simulink model "fft32kpt_ssr16_fixed"  (R2024b)
settings: Solver=VariableStepAuto  StartTime=0.0  StopTime=sample_period*N*5  RelTol=1e-3
PreLoadFcn:
  | clk_freq = 570e6; % PL clock frequency
  | sample_period = 1/(570e6*16); % 570Msps*16parallel paths
  | N=32768; % fft point size
  | binw=(1/sample_period) / 2*N; % bin width
  | 
  | bin_freq = 2*pi*11*binw+pi*binw; % sin, cos freq centering per channel
  | 
  | % for transpose block
  | DATA_WIDTH=16;
  | SSR=16;
  | M=16;
  | N1=N/M;
  | MEM_STYLE=4; % MEM OPTIONS: 4 - ULTRA, 0 - AUTO, 1 - BRAM, 5 - MIXED
InitFcn:
  | clk_freq = 570e6; % PL clock frequency
  | sample_period = 1/(570e6*16); % 570Msps*16parallel paths
  | N=32768; % fft point size
  | binw=(1/sample_period) / 2*N; % bin width
  | 
  | bin_freq = 2*pi*11*binw+pi*binw; % sin, cos freq centering per channel
  | 
  | % for transpose block
  | DATA_WIDTH=16;
  | SSR=16;
  | M=16;
  | N1=N/M;
  | MEM_STYLE=4; % MEM OPTIONS: 4 - ULTRA, 0 - AUTO, 1 - BRAM, 5 - MIXED
undefined symbols (not defined in the file or in its folder): None, S, vsva2197, xcvc1902
libraries: aieBasic x47, hdlBasic x39, aieUtilities x16, aieDSP x16, hdlUtilities x16, matrix_library x16, hdlSSR x13, simulink x1, dspxfrm3 x1, vmcUtilities x1
(part 3 of 3)

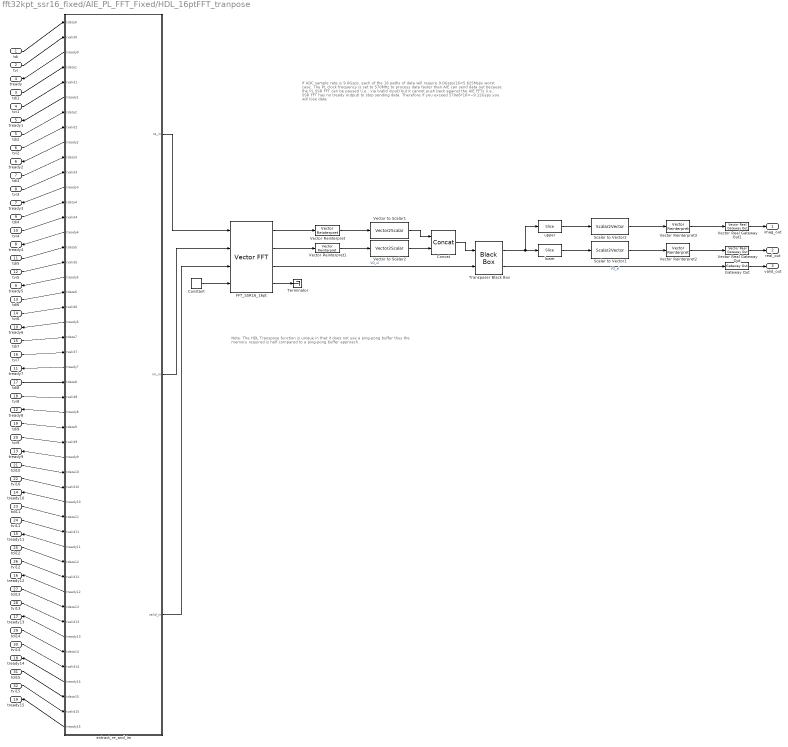
== system fft32kpt_ssr16_fixed/AIE_PL_FFT_Fixed/HDL_16ptFFT_tranpose ==
  note: If ADC sample rate is 9.0Gsps, each of the 16 paths of data will require 9.0Gsps/16=5.625Msps worst case. The PL clock frequency is set to 570MHz to process data faster than AIE can send data out because the PL SSR FFT can be paused (i.e.: via tvalid input) but it cannot push back against the AIE FFTs (i.e.: SSR FFT has no tready output) to stop sending data. Therefore if you exceed 570e6*16=~9.12Gsps you will lose data
  note: Note: The HDL Transpose function is unique in that it does not use a ping-pong buffer thus the memory required is half compared to a ping-pong buffer approach.
  tdi : Inport
  tvi : Inport  Port=2
  tdi1 : Inport  Port=3
  tvi1 : Inport  Port=4
  tdi2 : Inport  Port=5
  tvi2 : Inport  Port=6
  tdi3 : Inport  Port=7
  tvi3 : Inport  Port=8
  tdi4 : Inport  Port=9
  tvi4 : Inport  Port=10
  tdi5 : Inport  Port=11
  tvi5 : Inport  Port=12
  tdi6 : Inport  Port=13
  tvi6 : Inport  Port=14
  tdi7 : Inport  Port=15
  tvi7 : Inport  Port=16
  tdi8 : Inport  Port=17
  tvi8 : Inport  Port=18
  tdi9 : Inport  Port=19
  tvi9 : Inport  Port=20
  tdi10 : Inport  Port=21
  tvi10 : Inport  Port=22
  tdi11 : Inport  Port=23
  tvi11 : Inport  Port=24
  tdi12 : Inport  Port=25
  tvi12 : Inport  Port=26
  tdi13 : Inport  Port=27
  tvi13 : Inport  Port=28
  tdi14 : Inport  Port=29
  tvi14 : Inport  Port=30
  tdi15 : Inport  Port=31
  tvi15 : Inport  Port=32
  Concat : hdlBasic/Concat  num_inputs=2  XmcBlockStatus=1  maskContainerNames=group1  block_type=concat  block_config=sysgen:Concat_config
  Constant : hdlBasic/Constant  const=15  gui_display_data_type=Fixed-point  arith_type=Unsigned  n_bits=log2(16)  bin_pt=0  preci_type=Single  exp_width=8  frac_width=24  explicit_period=on  period=1/clk_freq  XmcBlockStatus=1  maskContainerNames=tabcontainer1  block_type=constant  block_config=sysgen:Constant_config
  FFT_SSR16_16pt : hdlSSR/Vector FFT  N=16  n_bits=16  bin_pt=0  rounding=on  bypass_input_swap=off  bypass_ouput_dsn=off  bram_threshold=258  use_cm4=3  use_cb=on  sg_ssr=16  block_type=fft_ssr  W_high=1  W_low=-17  XmcBlockStatus=1  sg_ssr_prev=16  maskContainerNames=group3
  Gateway Out : hdlBasic/Gateway Out  inherit_from_input=off  bool_to_boolean=off  hdl_port=on  rows=1  columns=1  UseAsDAC=off  DACChannel='1'  interface=None  automatic_assignment=on  address_offset=hex2dec('00')  intf_name=''  intf_description=''  timing_constraint=None  locs_specified=off  LOCs={}  io_standard={}  XmcBlockStatus=1  maskContainerNames=group4  block_type=gatewayout  block_config=sysgen:gateway_out_config  block_width_w=590  block_height_w=620  block_width=620  block_height=750
  Scalar to Vector1 : hdlSSR/Scalar2Vector  Width=DATA_WIDTH  sg_ssr=SSR  block_type=scalar2vector_ssr  XmcBlockStatus=1  sg_ssr_prev=16  maskContainerNames=group1
  Scalar to Vector2 : hdlSSR/Scalar2Vector  Width=DATA_WIDTH  sg_ssr=SSR  block_type=scalar2vector_ssr  XmcBlockStatus=1  sg_ssr_prev=16  maskContainerNames=group1
  Terminator : Terminator
  Transposer Black Box : hdlBasic/Black Box  init_code=ssr_transpose_top_config  sim_method=Vivado Simulator  engine_block=../../Questa  verbose=on  XmcBlockStatus=1  maskContainerNames=group1  block_type=blackbox2  block_config=sysgen:black_box_config
  Vector Real Gateway Out : hdlSSR/Vector Real Gateway Out  inherit_from_input=off  hdl_port=on  sg_ssr=16  rows=1  columns=1  UseAsDAC=off  DACChannel='1'  interface=None  automatic_assignment=on  address_offset=hex2dec('00')  intf_name=''  intf_description=''  timing_constraint=None  locs_specified=off  LOCs={}  io_standard={}  block_type=realgatewayout_ssr  XmcBlockStatus=1  sg_ssr_prev=16  maskContainerNames=group4  block_width_w=590  block_height_w=620  block_width=620  block_height=750
  Vector Real Gateway Out1 : hdlSSR/Vector Real Gateway Out  inherit_from_input=off  hdl_port=on  sg_ssr=16  rows=1  columns=1  UseAsDAC=off  DACChannel='1'  interface=None  automatic_assignment=on  address_offset=hex2dec('00')  intf_name=''  intf_description=''  timing_constraint=None  locs_specified=off  LOCs={}  io_standard={}  block_type=realgatewayout_ssr  XmcBlockStatus=1  sg_ssr_prev=16  maskContainerNames=group4  block_width_w=590  block_height_w=620  block_width=620  block_height=750
  Vector Reinterpret : hdlSSR/Vector Reinterpret  force_arith_type=on  arith_type=Unsigned  force_bin_pt=on  bin_pt=0  sg_ssr=SSR  block_type=reinterpret_ssr  XmcBlockStatus=1  sg_ssr_prev=16  maskContainerNames=group1
  Vector Reinterpret1 : hdlSSR/Vector Reinterpret  force_arith_type=on  arith_type=Unsigned  force_bin_pt=on  bin_pt=0  sg_ssr=SSR  block_type=reinterpret_ssr  XmcBlockStatus=1  sg_ssr_prev=16  maskContainerNames=group1
  Vector Reinterpret2 : hdlSSR/Vector Reinterpret  force_arith_type=on  arith_type="Signed  (2's comp)"  force_bin_pt=off  bin_pt=0  sg_ssr=SSR  block_type=reinterpret_ssr  XmcBlockStatus=1  sg_ssr_prev=16  maskContainerNames=group1
  Vector Reinterpret3 : hdlSSR/Vector Reinterpret  force_arith_type=on  arith_type="Signed  (2's comp)"  force_bin_pt=off  bin_pt=0  sg_ssr=SSR  block_type=reinterpret_ssr  XmcBlockStatus=1  sg_ssr_prev=16  maskContainerNames=group1
  Vector to Scalar1 : hdlSSR/Vector2Scalar  sg_ssr=SSR  block_type=vector2scalar_ssr  XmcBlockStatus=1  sg_ssr_prev=16  maskContainerNames=group1
  Vector to Scalar2 : hdlSSR/Vector2Scalar  sg_ssr=SSR  block_type=vector2scalar_ssr  XmcBlockStatus=1  sg_ssr_prev=16  maskContainerNames=group1
  extract_re_and_im : Subsystem
      settings: PortSchema="{\"entries\":[{\"content\":{\"sides\":[{\"content\":{\"connectorIds\":[\"In1\",\"In2\",\"Out4\",\"In3\",\"In4\",\"Out5\",\"In5\",\"In6\",\"Out6\",\"In7\",\"In8\",\"Out7\",\"In9\",\"In10\",\"Out8\",\"In11\",\"In12\",\"Out9\",\"In13\",\"In14\",\"Out10\",\"In15\",\"In16\",\"Out11\",\"In17\",\"In18\",\"Out12\",\"In19\",\"In20\",\"Out13\",\"In21\",\"In22\",\"Out14\",\"In23\",\"In24\",\"Out15\",\"In25\",\"In26\",\"Out16\",\"In27\",\"In28\",\"Out17\",\"In29\",\"In30\",\"Out18\",\"In31\",\"In32\",\"Out19\"]},\"type\":\"ConnectorPlacement.EquallySpacedRectSide\",\"uuid\":\"4c9cd091-c59a-490e-903e-02f0ef96851d\"},{\"content\":{\"connectorIds\":[\"Out1\",\"Out2\",\"Out3\"],\"side\":\"RIGHT\"},\"type\":\"ConnectorPlacement.EquallySpacedRectSide\",\"uuid\":\"c05feb9a-4f35-4110-be75-dac51685fe1e\"},{\"content\":{\"side\":\"TOP\"},\"type\":\"ConnectorPlacement.EquallySpacedRectSide\",\"uuid\":\"aa818d08-a3bb-44ec-b82c-f7b75f0c5c84\"}]},\"type\":\"ConnectorPlacement.EquallySpacedConnector\",\"uuid\":\"837a6877-8b4b-4e86-8a21-a8261c1d8bd7\"}],\"packageUris\":[\"http://schema.mathworks.com/mf0/Connector/R2020b\"],\"version\":\"1.0\"}"
  lower : hdlBasic/Slice  nbits=DATA_WIDTH*SSR  boolean_output=off  mode=Lower Bit Location + Width  bit1=0  base1=MSB of Input  bit0=0  base0=LSB of Input  XmcBlockStatus=1  maskContainerNames=group1  block_type=slice  block_config=sysgen:Slice_config
  upper : hdlBasic/Slice  nbits=DATA_WIDTH*SSR  boolean_output=off  mode=Upper Bit Location + Width  bit1=0  base1=MSB of Input  bit0=0  base0=LSB of Input  XmcBlockStatus=1  maskContainerNames=group1  block_type=slice  block_config=sysgen:Slice_config
  imag_out : Outport
  real_out : Outport  Port=2
  valid_out : Outport  Port=3
  tready : Outport  Port=4
  tready1 : Outport  Port=5
  tready2 : Outport  Port=6
  tready3 : Outport  Port=7
  tready4 : Outport  Port=8
  tready5 : Outport  Port=9
  tready6 : Outport  Port=10
  tready7 : Outport  Port=11
  tready8 : Outport  Port=12
  tready9 : Outport  Port=13
  tready10 : Outport  Port=14
  tready11 : Outport  Port=15
  tready12 : Outport  Port=16
  tready13 : Outport  Port=17
  tready14 : Outport  Port=18
  tready15 : Outport  Port=19
  wires:
  FFT_SSR16_16pt/4 -> Terminator/1
  Constant/1 -> FFT_SSR16_16pt/4
  extract_re_and_im/1(re_in) -> FFT_SSR16_16pt/1
  extract_re_and_im/2(im_in) -> FFT_SSR16_16pt/2
  tdi/1 -> extract_re_and_im/1(tdata0)
  tvi/1 -> extract_re_and_im/2(tvalid0)
  tdi1/1 -> extract_re_and_im/3(tdata1)
  tvi1/1 -> extract_re_and_im/4(tvalid1)
  tdi2/1 -> extract_re_and_im/5(tdata2)
  tvi2/1 -> extract_re_and_im/6(tvalid2)
  tdi3/1 -> extract_re_and_im/7(tdata3)
  tvi3/1 -> extract_re_and_im/8(tvalid3)
  tdi4/1 -> extract_re_and_im/9(tdata4)
  tvi4/1 -> extract_re_and_im/10(tvalid4)
  tdi5/1 -> extract_re_and_im/11(tdata5)
  tvi5/1 -> extract_re_and_im/12(tvalid5)
  tdi6/1 -> extract_re_and_im/13(tdata6)
  tvi6/1 -> extract_re_and_im/14(tvalid6)
  tdi7/1 -> extract_re_and_im/15(tdata7)
  tvi7/1 -> extract_re_and_im/16(tvalid7)
  tdi8/1 -> extract_re_and_im/17(tdata8)
  tvi8/1 -> extract_re_and_im/18(tvalid8)
  tdi9/1 -> extract_re_and_im/19(tdata9)
  tvi9/1 -> extract_re_and_im/20(tvalid9)
  tdi10/1 -> extract_re_and_im/21(tdata10)
  tvi10/1 -> extract_re_and_im/22(tvalid10)
  tdi11/1 -> extract_re_and_im/23(tdata11)
  tvi11/1 -> extract_re_and_im/24(tvalid11)
  tdi12/1 -> extract_re_and_im/25(tdata12)
  tvi12/1 -> extract_re_and_im/26(tvalid12)
  tdi13/1 -> extract_re_and_im/27(tdata13)
  tvi13/1 -> extract_re_and_im/28(tvalid13)
  tdi14/1 -> extract_re_and_im/29(tdata14)
  tvi14/1 -> extract_re_and_im/30(tvalid14)
  tdi15/1 -> extract_re_and_im/31(tdata15)
  tvi15/1 -> extract_re_and_im/32(tvalid15)
  extract_re_and_im/4(tready0) -> tready/1
  extract_re_and_im/5(tready1) -> tready1/1
  extract_re_and_im/6(tready2) -> tready2/1
  extract_re_and_im/3(valid_in) -> FFT_SSR16_16pt/3
  extract_re_and_im/7(tready3) -> tready3/1
  extract_re_and_im/8(tready4) -> tready4/1
  extract_re_and_im/9(tready5) -> tready5/1
  extract_re_and_im/10(tready6) -> tready6/1
  extract_re_and_im/11(tready7) -> tready7/1
  extract_re_and_im/12(tready8) -> tready8/1
  extract_re_and_im/13(tready9) -> tready9/1
  extract_re_and_im/14(tready10) -> tready10/1
  extract_re_and_im/15(tready11) -> tready11/1
  extract_re_and_im/16(tready12) -> tready12/1
  extract_re_and_im/17(tready13) -> tready13/1
  extract_re_and_im/18(tready14) -> tready14/1
  extract_re_and_im/19(tready15) -> tready15/1
  FFT_SSR16_16pt/2 -> Vector Reinterpret1/1
  FFT_SSR16_16pt/1 -> Vector Reinterpret/1
  FFT_SSR16_16pt/3 -> Transposer Black Box/2  "VO_sl"
  Vector Reinterpret2/1 -> Vector Real Gateway Out/1
  Vector Reinterpret3/1 -> Vector Real Gateway Out1/1
  Transposer Black Box/2 -> Gateway Out/1  "VO_sl"
  Vector to Scalar1/1 -> Concat/1
  Vector Reinterpret/1 -> Vector to Scalar1/1
  Scalar to Vector1/1 -> Vector Reinterpret2/1
  Transposer Black Box/1 -> upper/1, lower/1
  Vector to Scalar2/1 -> Concat/2
  lower/1 -> Scalar to Vector1/1
  Concat/1 -> Transposer Black Box/1
  upper/1 -> Scalar to Vector2/1
  Vector Reinterpret1/1 -> Vector to Scalar2/1
  Scalar to Vector2/1 -> Vector Reinterpret3/1
  Gateway Out/1 -> valid_out/1
  Vector Real Gateway Out/1 -> real_out/1
  Vector Real Gateway Out1/1 -> imag_out/1

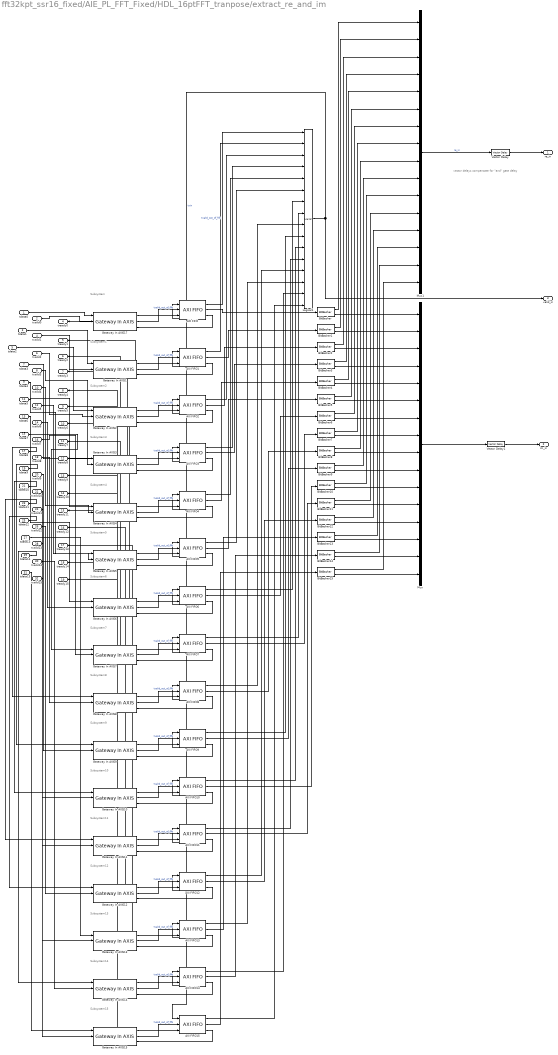
== system fft32kpt_ssr16_fixed/AIE_PL_FFT_Fixed/HDL_16ptFFT_tranpose/extract_re_and_im ==
  note: Subsystem15
  note: Subsystem14
  note: Subsystem13
  note: Subsystem12
  note: Subsystem11
  note: Subsystem10
  note: Subsystem9
  note: Subsystem8
  note: Subsystem7
  note: Subsystem6
  note: Subsystem5
  note: Subsystem4
  note: Subsystem3
  note: Subsystem2
  note: Subsystem1
  note: Subsystem
  note: vector delays compensate for "and" gate delay
  tdata0 : Inport
  tvalid0 : Inport  Port=2
  tdata1 : Inport  Port=3
  tvalid1 : Inport  Port=4
  tdata2 : Inport  Port=5
  tvalid2 : Inport  Port=6
  tdata3 : Inport  Port=7
  tvalid3 : Inport  Port=8
  tdata4 : Inport  Port=9
  tvalid4 : Inport  Port=10
  tdata5 : Inport  Port=11
  tvalid5 : Inport  Port=12
  tdata6 : Inport  Port=13
  tvalid6 : Inport  Port=14
  tdata7 : Inport  Port=15
  tvalid7 : Inport  Port=16
  tdata8 : Inport  Port=17
  tvalid8 : Inport  Port=18
  tdata9 : Inport  Port=19
  tvalid9 : Inport  Port=20
  tdata10 : Inport  Port=21
  tvalid10 : Inport  Port=22
  tdata11 : Inport  Port=23
  tvalid11 : Inport  Port=24
  tdata12 : Inport  Port=25
  tvalid12 : Inport  Port=26
  tdata13 : Inport  Port=27
  tvalid13 : Inport  Port=28
  tdata14 : Inport  Port=29
  tvalid14 : Inport  Port=30
  tdata15 : Inport  Port=31
  tvalid15 : Inport  Port=32
  AXI FIFO{,1..15} (16 alike) : hdlBasic/AXI FIFO  input_depth_axis=2K  actual_fifo_depth_label=2050  enable_tdata=on  enable_tdest=off  enable_tstrb=off  enable_tready=on  enable_tid=off  enable_tuser=off  enable_tkeep=off  enable_tlast=off  has_aresetn=off  enable_data_counts_axis=off  fifo_implementation_type_axis=Common Clock Block RAM  trim_axipin_name=on  programmable_full_type_axis=Full  full_threshold_assert_value_axis=0  programmable_empty_type_axis=Empty  empty_threshold_assert_value_axis=1022  underflow_flag_axi=0  underflow_sense_axi=Active High  overflow_flag_axi=0  overflow_sense_axi=Active High  simulation_type=fast_sim  XmcBlockStatus=1  maskContainerNames=tabcontainer1  block_type=axi_fifo  block_config=sysgen:AXI_FIFO_config
  BitBasher : hdlBasic/BitBasher  bitexpr=|  display_expr=off  sr_1=re  arith_type1="Signed  (2's comp)"  bin_pt1=0  sr_2=im  arith_type2="Signed  (2's comp)"  bin_pt2=0  sr_3=3  arith_type3=Unsigned  bin_pt3=0  sr_4=4  arith_type4=Unsigned  bin_pt4=0  XmcBlockStatus=1  maskContainerNames=group1  block_type=bitbasher  block_config=sysgen:BitBasher_config
      | re={inp[15:0]};
      | im={inp[31:16]};
  BitBasher1 : hdlBasic/BitBasher  bitexpr=|  display_expr=off  sr_1=re  arith_type1="Signed  (2's comp)"  bin_pt1=0  sr_2=im  arith_type2="Signed  (2's comp)"  bin_pt2=0  sr_3=3  arith_type3=Unsigned  bin_pt3=0  sr_4=4  arith_type4=Unsigned  bin_pt4=0  XmcBlockStatus=1  maskContainerNames=group1  block_type=bitbasher  block_config=sysgen:BitBasher_config
      | re={inp[15:0]};
      | im={inp[31:16]};
  BitBasher10 : hdlBasic/BitBasher  bitexpr=|  display_expr=off  sr_1=re  arith_type1="Signed  (2's comp)"  bin_pt1=0  sr_2=im  arith_type2="Signed  (2's comp)"  bin_pt2=0  sr_3=3  arith_type3=Unsigned  bin_pt3=0  sr_4=4  arith_type4=Unsigned  bin_pt4=0  XmcBlockStatus=1  maskContainerNames=group1  block_type=bitbasher  block_config=sysgen:BitBasher_config
      | re={inp[15:0]};
      | im={inp[31:16]};
  BitBasher11 : hdlBasic/BitBasher  bitexpr=|  display_expr=off  sr_1=re  arith_type1="Signed  (2's comp)"  bin_pt1=0  sr_2=im  arith_type2="Signed  (2's comp)"  bin_pt2=0  sr_3=3  arith_type3=Unsigned  bin_pt3=0  sr_4=4  arith_type4=Unsigned  bin_pt4=0  XmcBlockStatus=1  maskContainerNames=group1  block_type=bitbasher  block_config=sysgen:BitBasher_config
      | re={inp[15:0]};
      | im={inp[31:16]};
  BitBasher12 : hdlBasic/BitBasher  bitexpr=|  display_expr=off  sr_1=re  arith_type1="Signed  (2's comp)"  bin_pt1=0  sr_2=im  arith_type2="Signed  (2's comp)"  bin_pt2=0  sr_3=3  arith_type3=Unsigned  bin_pt3=0  sr_4=4  arith_type4=Unsigned  bin_pt4=0  XmcBlockStatus=1  maskContainerNames=group1  block_type=bitbasher  block_config=sysgen:BitBasher_config
      | re={inp[15:0]};
      | im={inp[31:16]};
  BitBasher13 : hdlBasic/BitBasher  bitexpr=|  display_expr=off  sr_1=re  arith_type1="Signed  (2's comp)"  bin_pt1=0  sr_2=im  arith_type2="Signed  (2's comp)"  bin_pt2=0  sr_3=3  arith_type3=Unsigned  bin_pt3=0  sr_4=4  arith_type4=Unsigned  bin_pt4=0  XmcBlockStatus=1  maskContainerNames=group1  block_type=bitbasher  block_config=sysgen:BitBasher_config
      | re={inp[15:0]};
      | im={inp[31:16]};
  BitBasher14 : hdlBasic/BitBasher  bitexpr=|  display_expr=off  sr_1=re  arith_type1="Signed  (2's comp)"  bin_pt1=0  sr_2=im  arith_type2="Signed  (2's comp)"  bin_pt2=0  sr_3=3  arith_type3=Unsigned  bin_pt3=0  sr_4=4  arith_type4=Unsigned  bin_pt4=0  XmcBlockStatus=1  maskContainerNames=group1  block_type=bitbasher  block_config=sysgen:BitBasher_config
      | re={inp[15:0]};
      | im={inp[31:16]};
  BitBasher15 : hdlBasic/BitBasher  bitexpr=|  display_expr=off  sr_1=re  arith_type1="Signed  (2's comp)"  bin_pt1=0  sr_2=im  arith_type2="Signed  (2's comp)"  bin_pt2=0  sr_3=3  arith_type3=Unsigned  bin_pt3=0  sr_4=4  arith_type4=Unsigned  bin_pt4=0  XmcBlockStatus=1  maskContainerNames=group1  block_type=bitbasher  block_config=sysgen:BitBasher_config
      | re={inp[15:0]};
      | im={inp[31:16]};
  BitBasher2 : hdlBasic/BitBasher  bitexpr=|  display_expr=off  sr_1=re  arith_type1="Signed  (2's comp)"  bin_pt1=0  sr_2=im  arith_type2="Signed  (2's comp)"  bin_pt2=0  sr_3=3  arith_type3=Unsigned  bin_pt3=0  sr_4=4  arith_type4=Unsigned  bin_pt4=0  XmcBlockStatus=1  maskContainerNames=group1  block_type=bitbasher  block_config=sysgen:BitBasher_config
      | re={inp[15:0]};
      | im={inp[31:16]};
  BitBasher3 : hdlBasic/BitBasher  bitexpr=|  display_expr=off  sr_1=re  arith_type1="Signed  (2's comp)"  bin_pt1=0  sr_2=im  arith_type2="Signed  (2's comp)"  bin_pt2=0  sr_3=3  arith_type3=Unsigned  bin_pt3=0  sr_4=4  arith_type4=Unsigned  bin_pt4=0  XmcBlockStatus=1  maskContainerNames=group1  block_type=bitbasher  block_config=sysgen:BitBasher_config
      | re={inp[15:0]};
      | im={inp[31:16]};
  BitBasher4 : hdlBasic/BitBasher  bitexpr=|  display_expr=off  sr_1=re  arith_type1="Signed  (2's comp)"  bin_pt1=0  sr_2=im  arith_type2="Signed  (2's comp)"  bin_pt2=0  sr_3=3  arith_type3=Unsigned  bin_pt3=0  sr_4=4  arith_type4=Unsigned  bin_pt4=0  XmcBlockStatus=1  maskContainerNames=group1  block_type=bitbasher  block_config=sysgen:BitBasher_config
      | re={inp[15:0]};
      | im={inp[31:16]};
  BitBasher5 : hdlBasic/BitBasher  bitexpr=|  display_expr=off  sr_1=re  arith_type1="Signed  (2's comp)"  bin_pt1=0  sr_2=im  arith_type2="Signed  (2's comp)"  bin_pt2=0  sr_3=3  arith_type3=Unsigned  bin_pt3=0  sr_4=4  arith_type4=Unsigned  bin_pt4=0  XmcBlockStatus=1  maskContainerNames=group1  block_type=bitbasher  block_config=sysgen:BitBasher_config
      | re={inp[15:0]};
      | im={inp[31:16]};
  BitBasher6 : hdlBasic/BitBasher  bitexpr=|  display_expr=off  sr_1=re  arith_type1="Signed  (2's comp)"  bin_pt1=0  sr_2=im  arith_type2="Signed  (2's comp)"  bin_pt2=0  sr_3=3  arith_type3=Unsigned  bin_pt3=0  sr_4=4  arith_type4=Unsigned  bin_pt4=0  XmcBlockStatus=1  maskContainerNames=group1  block_type=bitbasher  block_config=sysgen:BitBasher_config
      | re={inp[15:0]};
      | im={inp[31:16]};
  BitBasher7 : hdlBasic/BitBasher  bitexpr=|  display_expr=off  sr_1=re  arith_type1="Signed  (2's comp)"  bin_pt1=0  sr_2=im  arith_type2="Signed  (2's comp)"  bin_pt2=0  sr_3=3  arith_type3=Unsigned  bin_pt3=0  sr_4=4  arith_type4=Unsigned  bin_pt4=0  XmcBlockStatus=1  maskContainerNames=group1  block_type=bitbasher  block_config=sysgen:BitBasher_config
      | re={inp[15:0]};
      | im={inp[31:16]};
  BitBasher8 : hdlBasic/BitBasher  bitexpr=|  display_expr=off  sr_1=re  arith_type1="Signed  (2's comp)"  bin_pt1=0  sr_2=im  arith_type2="Signed  (2's comp)"  bin_pt2=0  sr_3=3  arith_type3=Unsigned  bin_pt3=0  sr_4=4  arith_type4=Unsigned  bin_pt4=0  XmcBlockStatus=1  maskContainerNames=group1  block_type=bitbasher  block_config=sysgen:BitBasher_config
      | re={inp[15:0]};
      | im={inp[31:16]};
  BitBasher9 : hdlBasic/BitBasher  bitexpr=|  display_expr=off  sr_1=re  arith_type1="Signed  (2's comp)"  bin_pt1=0  sr_2=im  arith_type2="Signed  (2's comp)"  bin_pt2=0  sr_3=3  arith_type3=Unsigned  bin_pt3=0  sr_4=4  arith_type4=Unsigned  bin_pt4=0  XmcBlockStatus=1  maskContainerNames=group1  block_type=bitbasher  block_config=sysgen:BitBasher_config
      | re={inp[15:0]};
      | im={inp[31:16]};
  Gateway In AXIS{1..15,17} (16 alike) : hdlUtilities/Gateway In AXIS  gui_display_data_type=Fixed-point  arith_type=Unsigned  n_bits=32  bin_pt=0  preci_type=Custom  exp_width=16  frac_width=24  quantization=Truncate  overflow=Wrap  bool_to_boolean=off  OutSampleTime=1/clk_freq  block_type=gatewayinaxi  XmcBlockStatus=1
  Logical1 : hdlBasic/Logical  logical_function=AND  inputs=16  en=off  latency=1  precision=Full  arith_type=Unsigned  n_bits=16  bin_pt=0  align_bp=on  overflow=[]  quantization=[]  XmcBlockStatus=1  maskContainerNames=tabcontainer1  block_type=logical  block_config=sysgen:Logical_config
  Mux : Mux  Inputs=16
  Mux1 : Mux  Inputs=16
  Vector Delay : hdlSSR/Vector Delay  rst=off  en=off  vectorize_en=off  sg_latency=1  sg_ssr=16  reg_retiming=off  block_type=delay_ssr  XmcBlockStatus=1  sg_ssr_prev=16  maskContainerNames=group1
  Vector Delay1 : hdlSSR/Vector Delay  rst=off  en=off  vectorize_en=off  sg_latency=1  sg_ssr=16  reg_retiming=off  block_type=delay_ssr  XmcBlockStatus=1  sg_ssr_prev=16  maskContainerNames=group1
  re_in : Outport
  im_in : Outport  Port=2
  valid_in : Outport  Port=3
  tready0 : Outport  Port=4
  tready1 : Outport  Port=5
  tready2 : Outport  Port=6
  tready3 : Outport  Port=7
  tready4 : Outport  Port=8
  tready5 : Outport  Port=9
  tready6 : Outport  Port=10
  tready7 : Outport  Port=11
  tready8 : Outport  Port=12
  tready9 : Outport  Port=13
  tready10 : Outport  Port=14
  tready11 : Outport  Port=15
  tready12 : Outport  Port=16
  tready13 : Outport  Port=17
  tready14 : Outport  Port=18
  tready15 : Outport  Port=19
  wires:
  BitBasher13/1 -> Mux1/14
  BitBasher15/2 -> Mux/16
  AXI FIFO7/2 -> BitBasher7/1
  BitBasher2/1 -> Mux1/3
  AXI FIFO14/1 -> Logical1/15
  Gateway In AXIS7/3 -> tready7/1
  AXI FIFO10/1 -> Logical1/11
  BitBasher14/1 -> Mux1/15
  AXI FIFO/1 -> Logical1/1  "tvalid_out_of_fifo"
  AXI FIFO6/1 -> Logical1/7
  AXI FIFO12/2 -> BitBasher12/1
  Gateway In AXIS13/3 -> tready13/1
  BitBasher/1 -> Mux1/1
  AXI FIFO8/1 -> Logical1/9
  BitBasher7/2 -> Mux/8
  BitBasher11/2 -> Mux/12
  BitBasher6/2 -> Mux/7
  AXI FIFO13/2 -> BitBasher13/1
  AXI FIFO5/1 -> Logical1/6
  BitBasher3/2 -> Mux/4
  AXI FIFO3/1 -> Logical1/4
  AXI FIFO1/1 -> Logical1/2
  BitBasher14/2 -> Mux/15
  BitBasher15/1 -> Mux1/16
  BitBasher1/1 -> Mux1/2
  BitBasher12/2 -> Mux/13
  AXI FIFO10/2 -> BitBasher10/1
  BitBasher12/1 -> Mux1/13
  BitBasher/2 -> Mux/1
  Gateway In AXIS10/3 -> tready10/1
  BitBasher9/2 -> Mux/10
  AXI FIFO4/2 -> BitBasher4/1
  Gateway In AXIS8/3 -> tready8/1
  Gateway In AXIS6/3 -> tready6/1
  Gateway In AXIS2/3 -> tready2/1
  BitBasher6/1 -> Mux1/7
  BitBasher5/2 -> Mux/6
  AXI FIFO2/1 -> Logical1/3
  Gateway In AXIS17/3 -> tready0/1
  Mux/1 -> Vector Delay1/1
  BitBasher3/1 -> Mux1/4
  Gateway In AXIS11/3 -> tready11/1
  BitBasher5/1 -> Mux1/6
  BitBasher4/1 -> Mux1/5
  AXI FIFO4/1 -> Logical1/5
  Gateway In AXIS12/3 -> tready12/1
  BitBasher7/1 -> Mux1/8
  AXI FIFO13/1 -> Logical1/14
  Gateway In AXIS3/3 -> tready3/1
  Gateway In AXIS1/3 -> tready1/1
  Logical1/1 -> valid_in/1, AXI FIFO/1, AXI FIFO1/1, AXI FIFO2/1, AXI FIFO3/1, AXI FIFO4/1, AXI FIFO5/1, AXI FIFO6/1, AXI FIFO7/1, AXI FIFO8/1, AXI FIFO9/1, AXI FIFO10/1, AXI FIFO11/1, AXI FIFO12/1, AXI FIFO13/1, AXI FIFO15/1, AXI FIFO14/1  "tvin"
  AXI FIFO11/2 -> BitBasher11/1
  AXI FIFO9/1 -> Logical1/10
  BitBasher10/1 -> Mux1/11
  Mux1/1 -> Vector Delay/1  "re_in"
  AXI FIFO14/2 -> BitBasher14/1
  Gateway In AXIS14/3 -> tready14/1
  AXI FIFO15/2 -> BitBasher15/1
  AXI FIFO15/1 -> Logical1/16
  BitBasher8/2 -> Mux/9
  AXI FIFO2/2 -> BitBasher2/1
  Gateway In AXIS4/3 -> tready4/1
  BitBasher8/1 -> Mux1/9
  BitBasher9/1 -> Mux1/10
  AXI FIFO5/2 -> BitBasher5/1
  AXI FIFO/2 -> BitBasher/1
  AXI FIFO12/1 -> Logical1/13
  BitBasher2/2 -> Mux/3
  Gateway In AXIS15/3 -> tready15/1
  BitBasher1/2 -> Mux/2
  Gateway In AXIS5/3 -> tready5/1
  AXI FIFO7/1 -> Logical1/8
  AXI FIFO11/1 -> Logical1/12
  AXI FIFO6/2 -> BitBasher6/1
  AXI FIFO3/2 -> BitBasher3/1
  BitBasher11/1 -> Mux1/12
  Gateway In AXIS9/3 -> tready9/1
  AXI FIFO1/2 -> BitBasher1/1
  BitBasher10/2 -> Mux/11
  AXI FIFO9/2 -> BitBasher9/1
  AXI FIFO8/2 -> BitBasher8/1
  BitBasher4/2 -> Mux/5
  BitBasher13/2 -> Mux/14
  Vector Delay/1 -> re_in/1
  Vector Delay1/1 -> im_in/1
  tdata0/1 -> Gateway In AXIS17/1
  AXI FIFO/3 -> Gateway In AXIS17/3
  tvalid0/1 -> Gateway In AXIS17/2
  Gateway In AXIS17/2 -> AXI FIFO/2  "tvalid_out_of_fifo"
  Gateway In AXIS17/1 -> AXI FIFO/3
  Gateway In AXIS1/1 -> AXI FIFO1/3
  Gateway In AXIS1/2 -> AXI FIFO1/2  "tvalid_out_of_fifo"
  tvalid1/1 -> Gateway In AXIS1/2
  AXI FIFO1/3 -> Gateway In AXIS1/3
  tdata1/1 -> Gateway In AXIS1/1
  tdata2/1 -> Gateway In AXIS2/1
  AXI FIFO2/3 -> Gateway In AXIS2/3
  tvalid2/1 -> Gateway In AXIS2/2
  Gateway In AXIS2/2 -> AXI FIFO2/2  "tvalid_out_of_fifo"
  Gateway In AXIS2/1 -> AXI FIFO2/3
  Gateway In AXIS3/1 -> AXI FIFO3/3
  Gateway In AXIS3/2 -> AXI FIFO3/2  "tvalid_out_of_fifo"
  tvalid3/1 -> Gateway In AXIS3/2
  AXI FIFO3/3 -> Gateway In AXIS3/3
  tdata3/1 -> Gateway In AXIS3/1
  Gateway In AXIS4/1 -> AXI FIFO4/3
  Gateway In AXIS4/2 -> AXI FIFO4/2  "tvalid_out_of_fifo"
  tvalid4/1 -> Gateway In AXIS4/2
  AXI FIFO4/3 -> Gateway In AXIS4/3
  tdata4/1 -> Gateway In AXIS4/1
  tdata5/1 -> Gateway In AXIS5/1
  AXI FIFO5/3 -> Gateway In AXIS5/3
  tvalid5/1 -> Gateway In AXIS5/2
  Gateway In AXIS5/2 -> AXI FIFO5/2  "tvalid_out_of_fifo"
  Gateway In AXIS5/1 -> AXI FIFO5/3
  Gateway In AXIS6/1 -> AXI FIFO6/3
  Gateway In AXIS6/2 -> AXI FIFO6/2  "tvalid_out_of_fifo"
  tvalid6/1 -> Gateway In AXIS6/2
  AXI FIFO6/3 -> Gateway In AXIS6/3
  tdata6/1 -> Gateway In AXIS6/1
  tdata7/1 -> Gateway In AXIS7/1
  AXI FIFO7/3 -> Gateway In AXIS7/3
  tvalid7/1 -> Gateway In AXIS7/2
  Gateway In AXIS7/2 -> AXI FIFO7/2  "tvalid_out_of_fifo"
  Gateway In AXIS7/1 -> AXI FIFO7/3
  Gateway In AXIS8/1 -> AXI FIFO8/3
  Gateway In AXIS8/2 -> AXI FIFO8/2  "tvalid_out_of_fifo"
  tvalid8/1 -> Gateway In AXIS8/2
  AXI FIFO8/3 -> Gateway In AXIS8/3
  tdata8/1 -> Gateway In AXIS8/1
  tdata9/1 -> Gateway In AXIS9/1
  AXI FIFO9/3 -> Gateway In AXIS9/3
  tvalid9/1 -> Gateway In AXIS9/2
  Gateway In AXIS9/2 -> AXI FIFO9/2  "tvalid_out_of_fifo"
  Gateway In AXIS9/1 -> AXI FIFO9/3
  Gateway In AXIS10/1 -> AXI FIFO10/3
  Gateway In AXIS10/2 -> AXI FIFO10/2  "tvalid_out_of_fifo"
  tvalid10/1 -> Gateway In AXIS10/2
  AXI FIFO10/3 -> Gateway In AXIS10/3
  tdata10/1 -> Gateway In AXIS10/1
  tdata11/1 -> Gateway In AXIS11/1
  AXI FIFO11/3 -> Gateway In AXIS11/3
  tvalid11/1 -> Gateway In AXIS11/2
  Gateway In AXIS11/2 -> AXI FIFO11/2  "tvalid_out_of_fifo"
  Gateway In AXIS11/1 -> AXI FIFO11/3
  tdata12/1 -> Gateway In AXIS12/1
  AXI FIFO12/3 -> Gateway In AXIS12/3
  tvalid12/1 -> Gateway In AXIS12/2
  Gateway In AXIS12/2 -> AXI FIFO12/2  "tvalid_out_of_fifo"
  Gateway In AXIS12/1 -> AXI FIFO12/3
  Gateway In AXIS13/1 -> AXI FIFO13/3
  Gateway In AXIS13/2 -> AXI FIFO13/2  "tvalid_out_of_fifo"
  tvalid13/1 -> Gateway In AXIS13/2
  AXI FIFO13/3 -> Gateway In AXIS13/3
  tdata13/1 -> Gateway In AXIS13/1
  tdata14/1 -> Gateway In AXIS14/1
  AXI FIFO14/3 -> Gateway In AXIS14/3
  tvalid14/1 -> Gateway In AXIS14/2
  Gateway In AXIS14/2 -> AXI FIFO14/2  "tvalid_out_of_fifo"
  Gateway In AXIS14/1 -> AXI FIFO14/3
  Gateway In AXIS15/1 -> AXI FIFO15/3
  Gateway In AXIS15/2 -> AXI FIFO15/2  "tvalid_out_of_fifo"
  tvalid15/1 -> Gateway In AXIS15/2
  AXI FIFO15/3 -> Gateway In AXIS15/3
  tdata15/1 -> Gateway In AXIS15/1
